simulink model "bird_eye_view_1"  (R2016a)
settings: Solver=VariableStepAuto  StartTime=0.0  StopTime=1  RelTol=1e-3
undefined symbols (not defined in the file): gray
libraries: visiongeotforms x2, visionsources x1
settings Model: Creator=Yewly  LastModifiedBy=Yewly

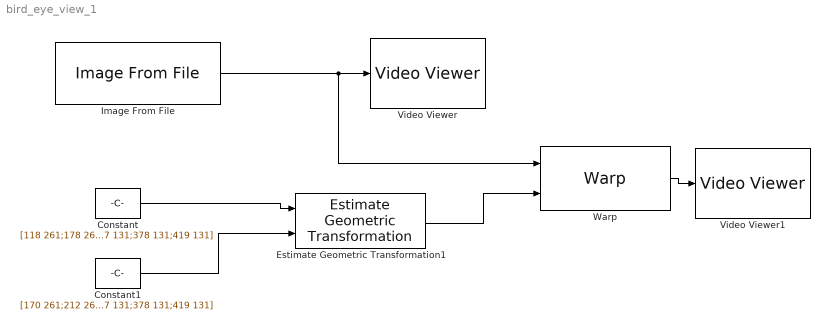
== system bird_eye_view_1 ==
  Constant : Constant  Value=[118 261;178 260;237 260;295 260;354 260;412 260;470 260;170 131;212 131;253 133;295 131;337 131;378 131;419 131]
  Constant1 : Constant  Value=[170 261;212 260;253 260;295 260 ;337 260;378 260;419 260;170 131;212 131;253 133;295 131;337 131;378 131;419 131]
  Estimate Geometric Transformation1 : visiongeotforms/Estimate Geometric Transformation  tformType=Projective  isRandomSampling=on  algMethod=Random Sample Consensus (RANSAC)  numMethod=Specified value  isStopSampling=off  percentStop=75  distanceAlg=2.5  distanceGeo=2.5  sampleNum=500  maxSampleNum=1000  desiredConfidence=99  isRefineTForm=off  isOutputInlier=off  outDT4IntInput=Obsolete10a  outDT4IntInputActive=Single  isVarSizeAllowed=on  isReleaseMode=on
  Image From File : visionsources/Image From File  Tag=vipblks_nd  FileName=chess2.jpg  imagePorts=One multidimensional signal  Ts=1  ImageDataType=Inherit from input image  Signed=on  WordLength=16  sdImageDataType=uint(8)  FractionLengthMode=User-defined  FractionLength=15  OutPortLabels=R|G|B
  Video Viewer : VideoViewer  colormapValue=gray(256)  FigPos=[381.8 654 552.8 396]
  Video Viewer1 : VideoViewer  colormapValue=gray(256)  FigPos=[823.4 664.4 544.8 394.4]
  Warp : visiongeotforms/Warp  TransformMatrixSource=Input port  TransformMatrix=eye( 3 )  InterpolationMethod=Bilinear  BackgroundFillValue=0  OutputImagePositionSource=Same as input image  OutputImagePosition=[ 1, 1, 512, 512 ]  ROIInputPort=off  ROIValidityOutputPort=off  SimulateUsing=Interpreted execution
  wires:
  Image From File/1 -> Warp/1, Video Viewer/1
  Estimate Geometric Transformation1/1 -> Warp/2
  Constant/1 -> Estimate Geometric Transformation1/1
  Constant1/1 -> Estimate Geometric Transformation1/2
  Warp/1 -> Video Viewer1/1
